simulink model "task_1"  (R2024a)
settings: Solver=FixedStepAuto  StartTime=0.0  StopTime=10  FixedStep=1e-5  RelTol=1e-3
undefined symbols (not defined in the file): a0, a1, idy, iy
settings Model: Creator=kit  LastModifiedBy=kit

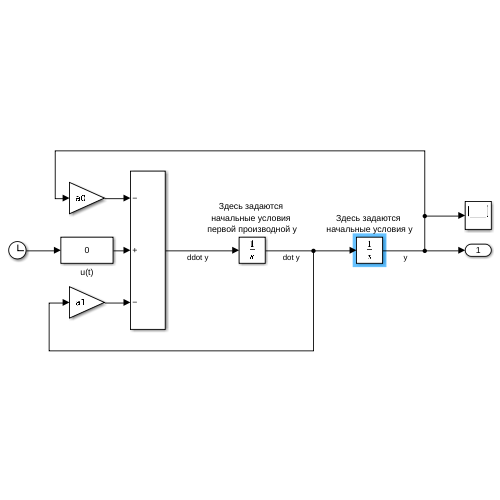
[thumbnail: Simulink's stored preview of the top-level diagram]
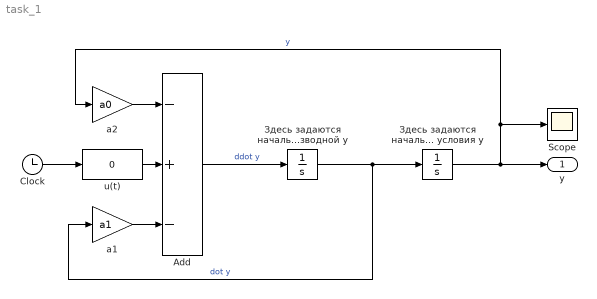
== system task_1 ==
  Add : Sum  Inputs=-+-
  Clock : Clock
  Scope : Scope
  a1 : Gain  Gain=a1
  a2 : Gain  Gain=a0
  u(t) : Fcn  Expr=0
  Здесь задаются начальные условия первой производной y : Integrator  InitialCondition=idy
  Здесь задаются начальные условия y : Integrator  InitialCondition=iy
  y : Outport
  wires:
  Clock/1 -> u(t)/1
  u(t)/1 -> Add/2
  a2/1 -> Add/1
  a1/1 -> Add/3
  Здесь задаются начальные условия первой производной y/1 -> a1/1, Здесь задаются начальные условия y/1  "dot y"
  Add/1 -> Здесь задаются начальные условия первой производной y/1  "ddot y"
  Здесь задаются начальные условия y/1 -> a2/1, Scope/1, y/1  "y"
